simulink model "DroneForwardingSimulation"  (R2022b)
settings: Solver=ode45  StartTime=0.0  StopTime=100  MaxStep=0.2  RelTol=1e-4  AbsTol=1e-4
libraries: slpidlib x1
settings Model: Creator=aless  LastModifiedBy=gianm

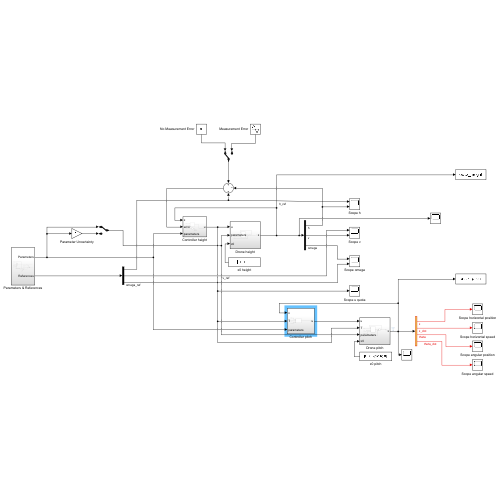
[thumbnail: Simulink's stored preview of the top-level diagram]
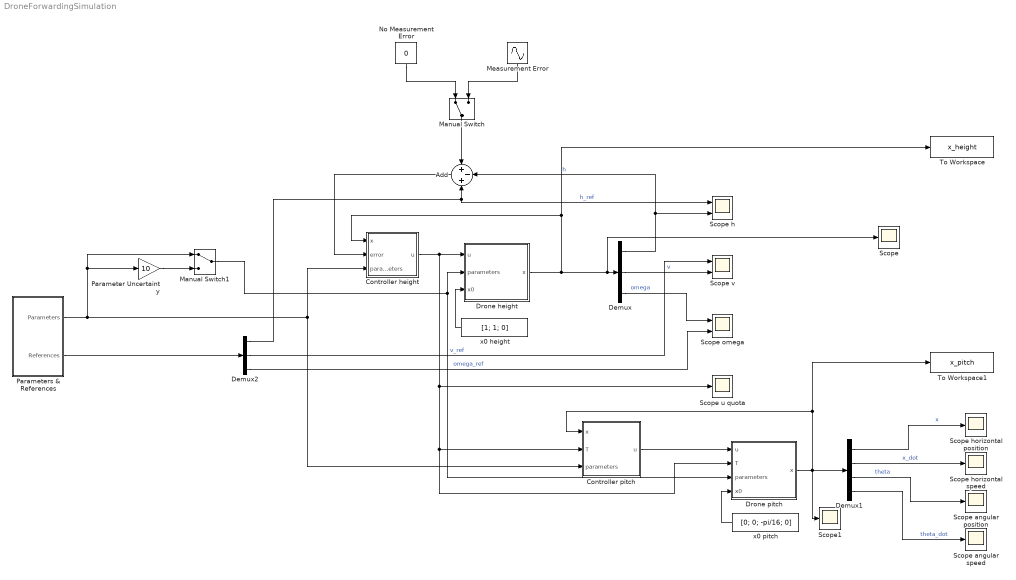
== system DroneForwardingSimulation ==
  Add : Sum  Inputs=+-+
  Controller height : Subsystem
  Controller pitch : Subsystem
  Demux : Demux  Outputs=3
  Demux1 : Demux
  Demux2 : Demux  Outputs=3
  Drone height : Subsystem
  Drone pitch : Subsystem
  Manual Switch : ManualSwitch
  Manual Switch1 : ManualSwitch
  Measurement Error : Sin  Frequency=0.1  SampleTime=0
  No Measurement Error : Constant  Value=0
  Parameter Uncertainty : Gain  Gain=10
  Parameters & References : Subsystem
  Scope : Scope
  Scope angular position : Scope
  Scope angular speed : Scope
  Scope h : Scope  NumInputPorts=2
  Scope horizontal position : Scope
  Scope horizontal speed : Scope
  Scope omega : Scope  NumInputPorts=2
  Scope u quota : Scope
  Scope v : Scope  NumInputPorts=2
  Scope1 : Scope
  To Workspace : ToWorkspace  VariableName=x_height  SaveFormat=Timeseries  SampleTime=0.1
  To Workspace1 : ToWorkspace  VariableName=x_pitch  SaveFormat=Timeseries  SampleTime=0.1
  x0 height : Constant  Value=[1; 1; 0]
  x0 pitch : Constant  Value=[0; 0; -pi/16; 0]
  wires:
  Drone height/1(x) -> To Workspace/1, Controller height/1(x), Scope/1, Demux/1
  Controller height/1(u) -> Scope u quota/1, Controller pitch/2(T), Drone pitch/2(T), Drone height/1(u)
  Demux/1 -> Add/2, Scope h/2  "h"
  Demux/2 -> Scope v/2  "v"
  Demux/3 -> Scope omega/1  "omega"
  x0 height/1 -> Drone height/3(x0)
  Add/1 -> Controller height/2(error)
  Controller pitch/1(u) -> Drone pitch/1(u)
  x0 pitch/1 -> Drone pitch/4(x0)
  Drone pitch/1(x) -> Scope1/1, Demux1/1, To Workspace1/1, Controller pitch/1(x)
  Demux1/1 -> Scope horizontal position/1  "x"
  Demux1/2 -> Scope horizontal speed/1  "x_dot"
  Demux1/3 -> Scope angular position/1  "theta"
  Demux1/4 -> Scope angular speed/1  "theta_dot"
  Parameters & References/2(References) -> Demux2/1
  Demux2/1 -> Scope h/1, Add/3  "h_ref"
  Demux2/2 -> Scope v/1  "v_ref"
  No Measurement Error/1 -> Manual Switch/1
  Measurement Error/1 -> Manual Switch/2
  Manual Switch/1 -> Add/1
  Parameters & References/1(Parameters) -> Controller height/3(parameters), Controller pitch/3(parameters), Parameter Uncertainty/1, Manual Switch1/1
  Parameter Uncertainty/1 -> Manual Switch1/2
  Manual Switch1/1 -> Drone pitch/3(parameters), Drone height/2(parameters)
  Demux2/3 -> Scope omega/2  "omega_ref"

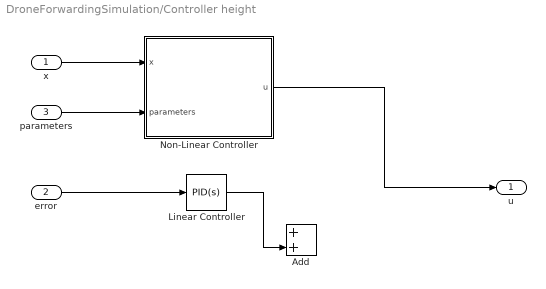
== system DroneForwardingSimulation/Controller height ==
  x : Inport
  error : Inport  Port=2
  parameters : Inport  Port=3
  Add : Sum
  Linear Controller : slpidlib/PID Controller  Controller=PID  Form=Parallel  TimeDomain=Continuous-time  UseExternalTs=off  SampleTime=-1  IntegratorMethod=Forward Euler  FilterMethod=Forward Euler  ControllerParametersSource=internal  P=20  I=5  UseKiTs=off  D=0  N=100  UseFilter=on  TunerSelectOption=Transfer Function Based (PID Tuner App)  InitialConditionSource=internal  InitialConditionForIntegrator=0  InitialConditionForFilter=0  DifferentiatorICPrevScaledInput=0  ExternalReset=none  TrackingMode=off  Kt=1  LimitOutput=off  SatLimitsSource=internal  UpperSaturationLimit=inf  LowerSaturationLimit=-inf  LinearizeAsGain=on  AntiWindupMode=none  Kb=1  LimitIntegrator=off  UpperIntegratorSaturationLimit=inf  LowerIntegratorSaturationLimit=-inf  POutMin=[]  POutMax=[]  IOutMin=[]  IOutMax=[]  DOutMin=[]  DOutMax=[]  NOutMin=[]  NOutMax=[]  SumOutMin=[]  SumOutMax=[]  SaturationOutMin=[]  SaturationOutMax=[]  PParamMin=[]  PParamMax=[]  IParamMin=[]  IParamMax=[]  DParamMin=[]  DParamMax=[]  NParamMin=[]  NParamMax=[]  KbParamMin=[]  KbParamMax=[]  KtParamMin=[]  KtParamMax=[]  KbOutMin=[]  KbOutMax=[]  KtOutMin=[]  KtOutMax=[]  IntegratorOutMin=[]  IntegratorOutMax=[]  FilterOutMin=[]  FilterOutMax=[]  SumI1OutMin=[]  SumI1OutMax=[]  SumI2OutMin=[]  SumI2OutMax=[]  SumI3OutMin=[]  SumI3OutMax=[]  SumI4OutMin=[]  SumI4OutMax=[]  SumDOutMin=[]  SumDOutMax=[]  DifferentiatorOutMin=[]  DifferentiatorOutMax=[]  FilterDiffOutCoefMin=[]  FilterDiffOutCoefMax=[]  ReciprocalOutMin=[]  ReciprocalOutMax=[]  SumDenOutMin=[]  SumDenOutMax=[]  SumNumOutMin=[]  SumNumOutMax=[]  DivideOutMin=[]  DivideOutMax=[]  UdiffTsProdOutMin=[]  UdiffTsProdOutMax=[]  NTsProdOutMin=[]  NTsProdOutMax=[]  UintegralTsProdOutMin=[]  UintegralTsProdOutMax=[]  UngainTsProdOutMin=[]  UngainTsProdOutMax=[]  ClampingZeroOutDataTypeStr=Inherit: Inherit via back propagation  ClampingZeroOutMin=[]  ClampingZeroOutMax=[]  FilterDenConstantOutDataTypeStr=Inherit: Inherit via back propagation  FilterDenConstantOutMin=[]  FilterDenConstantOutMax=[]  PCopyOutDataTypeStr=Inherit: Inherit via back propagation  PCopyOutMin=[]  PCopyOutMax=[]  NCopyOutDataTypeStr=Inherit: Inherit via back propagation  NCopyOutMin=[]  NCopyOutMax=[]  IntegratorContinuousStateAttributes=''  IntegratorStateMustResolveToSignalObject=off  IntegratorRTWStateStorageClass=Auto  FilterContinuousStateAttributes=''  FilterStateMustResolveToSignalObject=off  FilterRTWStateStorageClass=Auto  ParallelPVariant=InternalParameters  IdealPVariant=Disabled  IVariant=InternalParameters  DVariant=InternalParameters  IntegratorVariant=Continuous  SatVariant=Disabled  AWVariant=Passthrough  PCopyVariant=Disabled  TRVariant=Disabled  FdbkBlocksVariant=Forward  IdealPFdbkVariant=Disabled  SatFdbkVariant=Disabled  DerivativeFilterVariant=ContFilter  NVariant=InternalParameters  NCopyVariant=Disabled  FilterICVariant=InternalICsFilter  IntegratorICVariant=InternalICs  ExternalResetVariant=Disabled  TRSumVariant=Passthrough  SumFdbkVariant=Disabled  SumVariant=Sum_PID  TsampFilterVariant=InternalTs  TsampNgainVariant=Passthrough  TsampIntegralVariant=Passthrough  ExternalSaturationOutDataTypeStr=Inherit: Same as second input
  Non-Linear Controller : MATLAB Function  TreatAsAtomicUnit=on
  u : Outport
  wires:
  parameters/1 -> Non-Linear Controller/2(parameters)
  x/1 -> Non-Linear Controller/1(x)
  error/1 -> Linear Controller/1
  Non-Linear Controller/1(u) -> u/1
  Linear Controller/1 -> Add/2

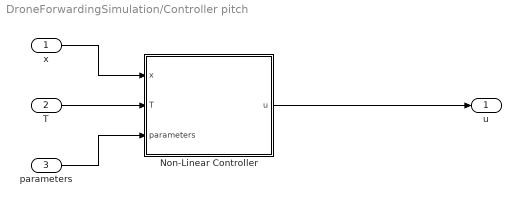
== system DroneForwardingSimulation/Controller pitch ==
  x : Inport
  T : Inport  Port=2
  parameters : Inport  Port=3
  Non-Linear Controller : MATLAB Function  TreatAsAtomicUnit=on
  u : Outport
  wires:
  parameters/1 -> Non-Linear Controller/3(parameters)
  x/1 -> Non-Linear Controller/1(x)
  Non-Linear Controller/1(u) -> u/1
  T/1 -> Non-Linear Controller/2(T)

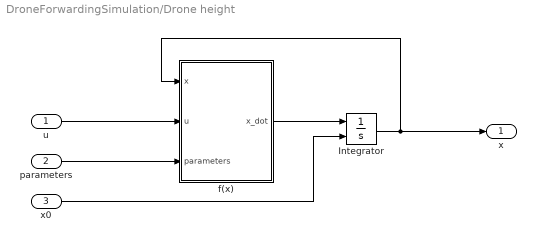
== system DroneForwardingSimulation/Drone height ==
  u : Inport
  parameters : Inport  Port=2
  x0 : Inport  Port=3
  Integrator : Integrator  InitialConditionSource=external
  f(x) : MATLAB Function  TreatAsAtomicUnit=on
  x : Outport
  wires:
  Integrator/1 -> x/1, f(x)/1(x)
  f(x)/1(x_dot) -> Integrator/1
  u/1 -> f(x)/2(u)
  parameters/1 -> f(x)/3(parameters)
  x0/1 -> Integrator/2

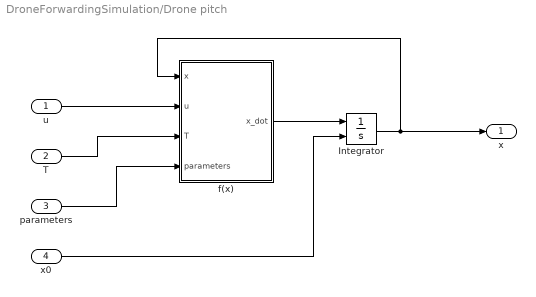
== system DroneForwardingSimulation/Drone pitch ==
  u : Inport
  T : Inport  Port=2
  parameters : Inport  Port=3
  x0 : Inport  Port=4
  Integrator : Integrator  InitialConditionSource=external
  f(x) : MATLAB Function  TreatAsAtomicUnit=on
  x : Outport
  wires:
  Integrator/1 -> x/1, f(x)/1(x)
  f(x)/1(x_dot) -> Integrator/1
  u/1 -> f(x)/2(u)
  parameters/1 -> f(x)/4(parameters)
  x0/1 -> Integrator/2
  T/1 -> f(x)/3(T)

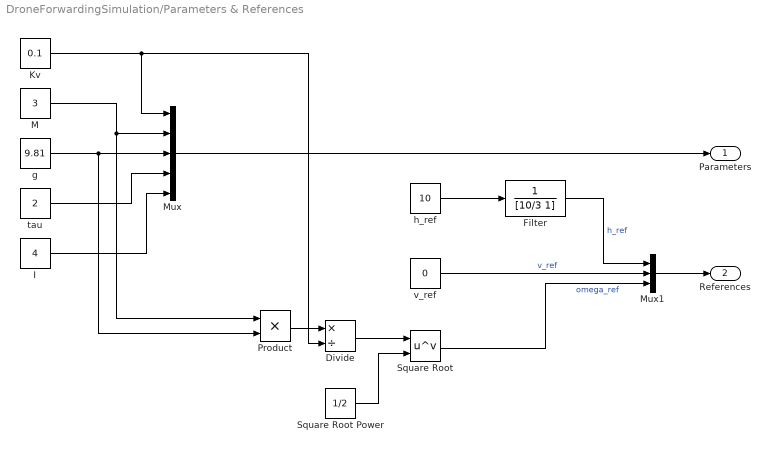
== system DroneForwardingSimulation/Parameters & References ==
  Divide : Product  Inputs=*/
  Filter : TransferFcn  Denominator=[10/3 1]
  I : Constant  Value=4
  Kv : Constant  Value=0.1
  M : Constant  Value=3
  Mux : Mux  Inputs=5
  Mux1 : Mux  Inputs=3
  Product : Product
  Square Root : Math  Operator=pow
  Square Root Power : Constant  Value=1/2
  g : Constant  Value=9.81
  h_ref : Constant  Value=10
  tau : Constant  Value=2
  v_ref : Constant  Value=0
  Parameters : Outport
  References : Outport  Port=2
  wires:
  g/1 -> Product/2, Mux/3
  Kv/1 -> Divide/2, Mux/1
  tau/1 -> Mux/4
  M/1 -> Product/1, Mux/2
  Mux/1 -> Parameters/1
  Divide/1 -> Square Root/1
  Square Root Power/1 -> Square Root/2
  Product/1 -> Divide/1
  I/1 -> Mux/5
  h_ref/1 -> Filter/1
  Filter/1 -> Mux1/1  "h_ref"
  Mux1/1 -> References/1
  v_ref/1 -> Mux1/2  "v_ref"
  Square Root/1 -> Mux1/3  "omega_ref"

== matlab function DroneForwardingSimulation/Controller height/Non-Linear Controller ==
  data: x input; u output; parameters input
function u = fcn(x, parameters)

    Kv =    parameters(1);
    M =     parameters(2);
    g =     parameters(3);
    tau =   parameters(4);
    x1 = x(1);
    x3 = x(3);
    x2 = x(2);
    a = 2*Kv/M *sqrt(M/Kv *g);

    u = -(x3 + (x2 + Kv/M * tau/2 *x3^2 + tau*a*x3)*(Kv*tau/M * x3 + tau*a))+...
    -x3 - (1/(8*a^3*tau^2*(1 + 2*tau)^2*(1 + tau + a^2*tau^3)^2)) * ...
    (2 + 2*a^4*tau^5 + a^2*tau^3*(4 + Kv*M*x2) + a^3*Kv*M*tau^4*x3 + ...
    2*a*tau^2*(a + Kv*M*x3) + tau*(2 + a*Kv*M*x3)) * ...
    (-4*(1 + tau)^2*x2 + 4*a^5*tau^7*x3 + 4*a*tau^2*(1 + tau)*x3 + ...
    2*a^3*tau^4*(2 + tau*(4 + Kv*M*x2))*x3 + ...
    a^4*tau^5*(4*x1 + 8*tau*x1 + 4*tau*x2 + Kv*M*tau*x3^2) + ...
    a^2*tau^2*(4*(1 + 3*tau + 2*tau^2)*x1 + ...
    Kv*M*tau*(tau*x2^2 + x3^2 + 2*tau*x3^2))) - ...
    (a*tau + (Kv*x3)/M) * ...
    (x2 + ((-2 - 4*tau - 2*tau^2 + 2*a^4*tau^6 + a^2*Kv*M*tau^4*x2 + ...
    a^3*Kv*M*tau^5*x3) * ...
    (-4*(1 + tau)^2*x2 + 4*a^5*tau^7*x3 + ...
    4*a*tau^2*(1 + tau)*x3 + ...
    2*a^3*tau^4*(2 + tau*(4 + Kv*M*x2))*x3 + ...
    a^4*tau^5*(4*x1 + 8*tau*x1 + 4*tau*x2 + Kv*M*tau*x3^2) + ...
    a^2*tau^2*(4*(1 + 3*tau + 2*tau^2)*x1 + ...
    Kv*M*tau*(tau*x2^2 + x3^2 + 2*tau*x3^2)))) / ...
    (8*a^4*tau^4*(1 + 2*tau)^2*(1 + tau + a^2*tau^3)^2));

end

== matlab function DroneForwardingSimulation/Drone height/f(x) ==
  data: x input; u input; x_dot output; parameters input
function x_dot = fcn(x, u, parameters)

    Kv =    parameters(1);
    M =     parameters(2);
    g =     parameters(3);
    tau =   parameters(4);
    a = 2*Kv/M *sqrt(M/Kv *g);

    x_dot = [x(2);
            (Kv/M)*x(3)^2 + a*x(3);
            (-x(3)/tau +u)];

end

== matlab function DroneForwardingSimulation/Drone pitch/f(x) ==
  data: x input; u input; T input; x_dot output; parameters input
function x_dot = fcn(x, u, T, parameters)

    M =     parameters(2);
    I =     parameters(5);

    x_dot = [+x(2);
             -T/M * sin(x(3));
             +x(4);
             -x(4)+ u];

end

== matlab function DroneForwardingSimulation/Controller pitch/Non-Linear Controller ==
  data: x input; T input; u output; parameters input
function u = fcn(x, T, parameters)

    M =     parameters(2);
    I =     parameters(5);

%     u0 = - x(4);
% 
%     u1 = - (x(4) + (x(3) + I*x(4)) * I) * 1/I;
% 
%     u2 = - (x(4) - (x(2) - T/M * (I^2*x(4) - I^4*x(4)^3/18) * T/M * (I^2 - I^4*x(4)^2/6))) * 1/I;   

    % u3 = - (x(4) + (x(1) + T/M * (I^3*x(4) - I^5*x(4)^3/48) * T/M * (I^3 - I^5*x(4)^2/18))) * 1/I;
    x2 = x(2);
    x3 = x(3);
    x4 = x(4);
    v = -(x3 + 2*x4);
    v2 = -x3 - 2*x4 + (T*(x3 + x4)*(684 - 84*x4^2 + 222*x4*(x3 + x4) - 150*(x3 + x4)^2))/(342*M) ...
    + (T*(x3 + x4)*(-300*x4*(x3 + x4) + 207*(x3 + x4)^2 + 3*(-342 + 37*x4^2)))/(342*M);


    
    u = v + v2;

end
